simulink subsystem "DR"  (R2024a)
settings: Solver=VariableStepAuto  StartTime=0.0  StopTime=200.0  RelTol=1e-3
undefined symbols (not defined in the file): MBS_deltaFrontSlant, MBS_deltaRearSlant
settings Model: DefaultTestHarness=DR_Harness  Creator=nicol  LastModifiedBy=nicol

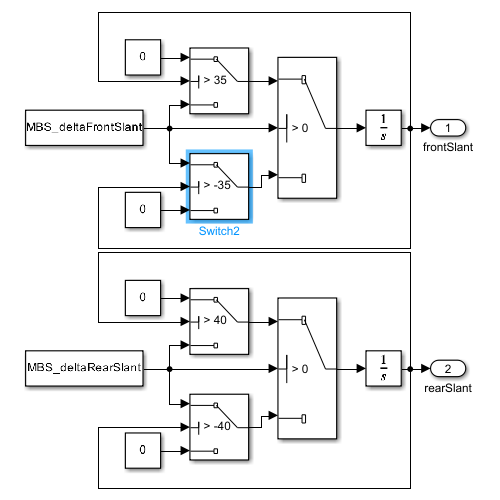
[thumbnail: Simulink's stored preview of the top-level diagram]
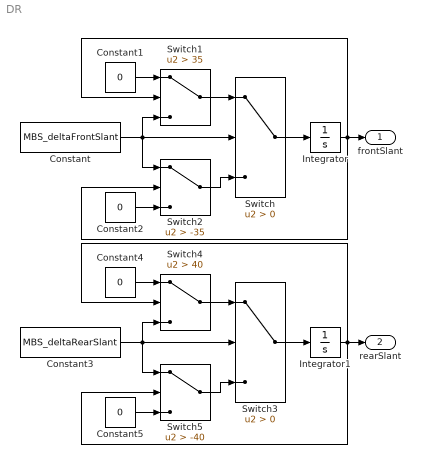
== system DR ==
  Constant : Constant  Value=MBS_deltaFrontSlant
  Constant{1..2,4..5} (4 alike) : Constant  Value=0
  Constant3 : Constant  Value=MBS_deltaRearSlant
  Integrator : Integrator
  Integrator1 : Integrator
  Switch : Switch  Criteria=u2 > Threshold  SaturateOnIntegerOverflow=off  InputSameDT=off
  Switch1 : Switch  Criteria=u2 > Threshold  Threshold=35  SaturateOnIntegerOverflow=off  InputSameDT=off
  Switch2 : Switch  Criteria=u2 > Threshold  Threshold=-35  SaturateOnIntegerOverflow=off  InputSameDT=off
  Switch3 : Switch  Criteria=u2 > Threshold  SaturateOnIntegerOverflow=off  InputSameDT=off
  Switch4 : Switch  Criteria=u2 > Threshold  Threshold=40  SaturateOnIntegerOverflow=off  InputSameDT=off
  Switch5 : Switch  Criteria=u2 > Threshold  Threshold=-40  SaturateOnIntegerOverflow=off  InputSameDT=off
  frontSlant : Outport
  rearSlant : Outport  Port=2
  wires:
  Integrator/1 -> Switch1/2, Switch2/2, frontSlant/1
  Switch1/1 -> Switch/1
  Switch2/1 -> Switch/3
  Constant/1 -> Switch1/3, Switch2/1, Switch/2
  Switch/1 -> Integrator/1
  Constant2/1 -> Switch2/3
  Constant1/1 -> Switch1/1
  Integrator1/1 -> rearSlant/1, Switch4/2, Switch5/2
  Constant3/1 -> Switch4/3, Switch5/1, Switch3/2
  Switch5/1 -> Switch3/3
  Constant5/1 -> Switch5/3
  Switch4/1 -> Switch3/1
  Switch3/1 -> Integrator1/1
  Constant4/1 -> Switch4/1
